simulink model "Week7"  (R2022a)
settings: Solver=ode4  StartTime=0.0  StopTime=10.0  RelTol=1e-3
values from neighbouring files (symbols this model uses):
  G1 = 7.77777777778    [Constants.mat]
  G2 = -2    [Constants.mat]
  tou = 0.5    [Constants.mat]
settings Model: Creator=Josh2  LastModifiedBy=Josh2

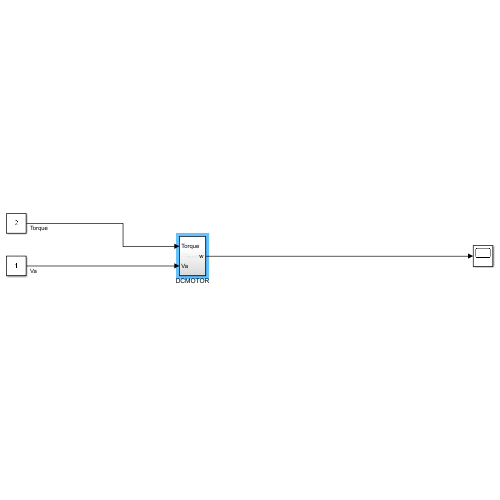
[thumbnail: Simulink's stored preview of the top-level diagram]
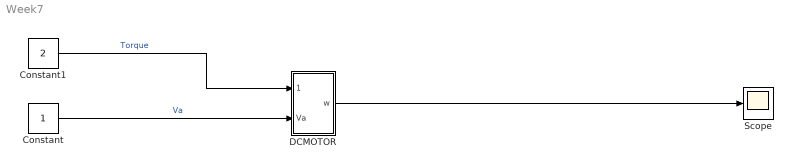
== system Week7 ==
  Constant : Constant
  Constant1 : Constant  Value=2
  DCMOTOR : Subsystem
  Scope : Scope
  wires:
  Constant1/1 -> DCMOTOR/1(Torque)  "Torque"
  Constant/1 -> DCMOTOR/2(Va)  "Va"
  DCMOTOR/1(w) -> Scope/1

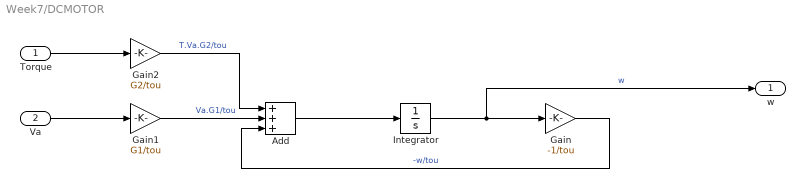
== system Week7/DCMOTOR ==
  Torque : Inport
  Va : Inport  Port=2
  Add : Sum  Inputs=+++
  Gain : Gain  Gain=-1/tou
  Gain1 : Gain  Gain=G1/tou
  Gain2 : Gain  Gain=G2/tou
  Integrator : Integrator
  w : Outport
  wires:
  Gain1/1 -> Add/2  "Va.G1/tou"
  Gain2/1 -> Add/1  "T.Va.G2/tou"
  Va/1 -> Gain1/1
  Integrator/1 -> w/1, Gain/1  "w"
  Add/1 -> Integrator/1
  Gain/1 -> Add/3  "-w/tou"
  Torque/1 -> Gain2/1
